simulink model "test"  (R2025a)
settings: Solver=VariableStepAuto  StartTime=0.0  StopTime=10.0  RelTol=1e-3
settings Model: Creator=josephderay  LastModifiedBy=josephderay

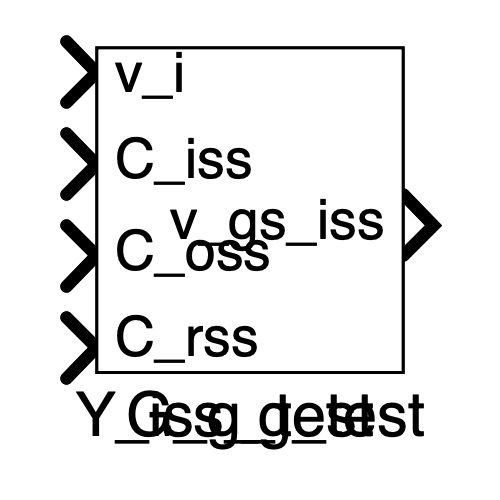
[thumbnail: Simulink's stored preview of the top-level diagram]
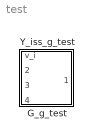
== system test ==
  G_g_test : Subsystem
  Y_iss_g_test : Subsystem

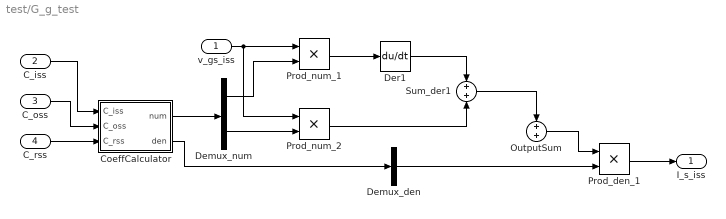
== system test/G_g_test ==
  v_gs_iss : Inport
  C_iss : Inport  Port=2
  C_oss : Inport  Port=3
  C_rss : Inport  Port=4
  CoeffCalculator : MATLAB Function  TreatAsAtomicUnit=on
  Demux_den : Demux  Outputs=1
  Demux_num : Demux  Outputs=2
  Der1 : Derivative
  OutputSum : Sum
  Prod_den_1 : Product
  Prod_num_1 : Product
  Prod_num_2 : Product
  Sum_der1 : Sum
  I_s_iss : Outport
  wires:
  Sum_der1/1 -> OutputSum/1
  OutputSum/1 -> Prod_den_1/1
  Demux_den/1 -> Prod_den_1/2
  Prod_num_1/1 -> Der1/1
  Prod_den_1/1 -> I_s_iss/1
  v_gs_iss/1 -> Prod_num_2/1, Prod_num_1/1
  Demux_num/1 -> Prod_num_1/2
  CoeffCalculator/2(den) -> Demux_den/1
  Der1/1 -> Sum_der1/1
  Prod_num_2/1 -> Sum_der1/2
  C_oss/1 -> CoeffCalculator/2(C_oss)
  Demux_num/2 -> Prod_num_2/2
  C_iss/1 -> CoeffCalculator/1(C_iss)
  CoeffCalculator/1(num) -> Demux_num/1
  C_rss/1 -> CoeffCalculator/3(C_rss)

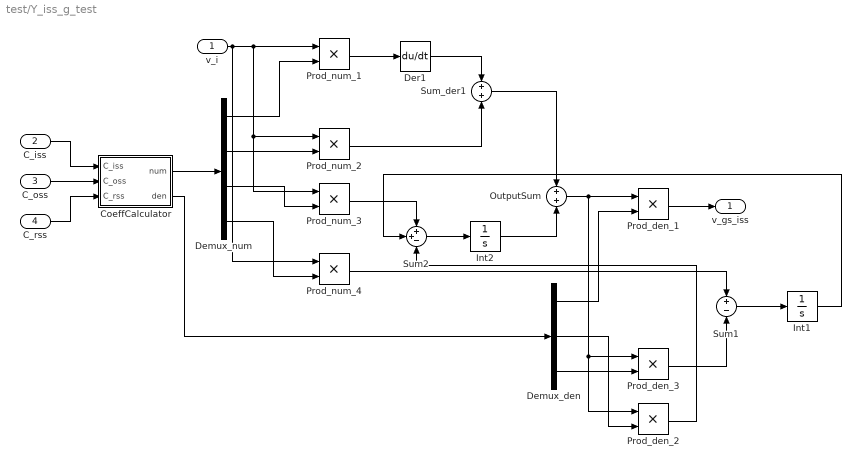
== system test/Y_iss_g_test ==
  v_i : Inport
  C_iss : Inport  Port=2
  C_oss : Inport  Port=3
  C_rss : Inport  Port=4
  CoeffCalculator : MATLAB Function  TreatAsAtomicUnit=on
  Demux_den : Demux  Outputs=3
  Demux_num : Demux
  Der1 : Derivative
  Int1 : Integrator
  Int2 : Integrator
  OutputSum : Sum
  Prod_den_1 : Product
  Prod_den_2 : Product
  Prod_den_3 : Product
  Prod_num_{1..4} (4 alike) : Product
  Sum1 : Sum  Inputs=+-
  Sum2 : Sum  Inputs=++-
  Sum_der1 : Sum
  v_gs_iss : Outport
  wires:
  Int1/1 -> Sum2/2
  Sum1/1 -> Int1/1
  Prod_den_2/1 -> Sum2/3
  Prod_num_4/1 -> Sum1/1
  Demux_den/3 -> Prod_den_3/2
  v_i/1 -> Prod_num_3/1, Prod_num_2/1, Prod_num_1/1, Prod_num_4/1
  Prod_den_1/1 -> v_gs_iss/1
  Int2/1 -> OutputSum/2
  Demux_den/2 -> Prod_den_2/2
  OutputSum/1 -> Prod_den_3/1, Prod_den_2/1, Prod_den_1/1
  Prod_num_2/1 -> Sum_der1/2
  Prod_num_1/1 -> Der1/1
  Demux_den/1 -> Prod_den_1/2
  Demux_num/4 -> Prod_num_4/2
  Sum2/1 -> Int2/1
  Demux_num/2 -> Prod_num_2/2
  Der1/1 -> Sum_der1/1
  Prod_num_3/1 -> Sum2/1
  Demux_num/1 -> Prod_num_1/2
  CoeffCalculator/1(num) -> Demux_num/1
  C_rss/1 -> CoeffCalculator/3(C_rss)
  Sum_der1/1 -> OutputSum/1
  C_iss/1 -> CoeffCalculator/1(C_iss)
  CoeffCalculator/2(den) -> Demux_den/1
  Prod_den_3/1 -> Sum1/2
  Demux_num/3 -> Prod_num_3/2
  C_oss/1 -> CoeffCalculator/2(C_oss)

== matlab function test/G_g_test/CoeffCalculator ==
  data: C_iss input; num output; C_oss input; C_rss input; den output
function [num,den] = CoeffCalculator(C_iss,C_oss,C_rss)
%#codegen

%    This function was generated by the Symbolic Math Toolbox version 25.1.
%    31-Jul-2025 12:28:13

% C_iss = complex(C_iss);  % if required to enforce complex operations
% C_oss = complex(C_oss);  % if required to enforce complex operations
% C_rss = complex(C_rss);  % if required to enforce complex operations
num = [C_iss-C_rss,0.0];
if nargout > 1
    den = 1.0;
end
end

== matlab function test/Y_iss_g_test/CoeffCalculator ==
  data: C_iss input; num output; C_oss input; C_rss input; den output
function [num,den] = CoeffCalculator(C_iss,C_oss,C_rss)
%#codegen

%    This function was generated by the Symbolic Math Toolbox version 25.1.
%    31-Jul-2025 12:29:46

% C_iss = complex(C_iss);  % if required to enforce complex operations
% C_oss = complex(C_oss);  % if required to enforce complex operations
% C_rss = complex(C_rss);  % if required to enforce complex operations
t2 = C_oss.*1.0e+9;
num = [1.0,1.0,t2,2.00000001e+8];
if nargout > 1
    den = [C_rss.^2.*-5.0e+9+C_iss.*C_oss.*5.0e+9,C_iss.*1.000000005e+9+t2,2.00000001e+8];
end
end
